simulink model "oppg1_system"  (R2014b)
settings: Solver=ode45  StartTime=0.0  StopTime=10  FixedStep=0.1  RelTol=1e-3
values from neighbouring files (symbols this model uses):
  A = 1    [main_1.m]    (also in main_tau.m)
  h_0 = 0    [main_1.m]    (also in main_tau.m)
  h_r = 0.5    [main_1.m]    (also in main_tau.m)
  k = 1    [main_1.m]    (also in main_tau.m)
  k_i = 0.1    [main_1.m]    (also in main_tau.m = 4)
  k_p = 100    [main_1.m]    (also in main_tau.m)
  rho = 1000    [main_1.m]    (also in main_tau.m)
  tau = 0    [main_1.m]    (also in main_tau.m = tau_list(i))
  w_f = 10    [main_1.m]    (also in main_tau.m = 0)
settings Model: Creator=rende_000  LastModifiedBy=rende_000

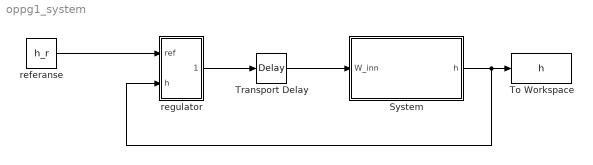
== system oppg1_system ==
  System : Subsystem
  To Workspace : ToWorkspace  VariableName=h  SaveFormat=Timeseries  SampleTime=-1
  Transport Delay : TransportDelay  DelayTime=tau
  referanse : Constant  Value=h_r
  regulator : Subsystem
  wires:
  System/1(h) -> regulator/2(h), To Workspace/1
  referanse/1 -> regulator/1(ref)
  regulator/1(Pådrag) -> Transport Delay/1
  Transport Delay/1 -> System/1(W_inn)

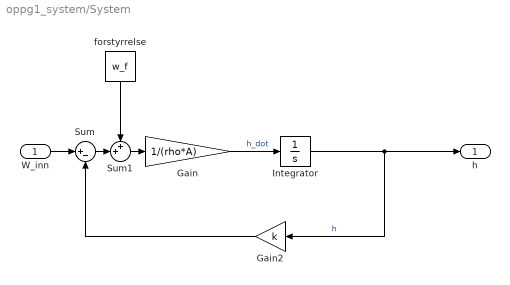
== system oppg1_system/System ==
  W_inn : Inport
  Gain : Gain  Gain=1/(rho*A)
  Gain2 : Gain  Gain=k
  Integrator : Integrator  InitialCondition=h_0
  Sum : Sum  Inputs=|+-
  Sum1 : Sum  Inputs=++|
  forstyrrelse : Constant  Value=w_f
  h : Outport
  wires:
  Gain2/1 -> Sum/2
  Integrator/1 -> h/1, Gain2/1  "h"
  Gain/1 -> Integrator/1  "h_dot"
  W_inn/1 -> Sum/1
  Sum1/1 -> Gain/1
  Sum/1 -> Sum1/2
  forstyrrelse/1 -> Sum1/1

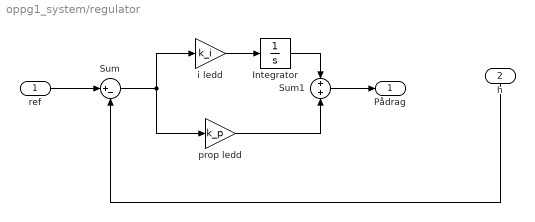
== system oppg1_system/regulator ==
  ref : Inport
  h : Inport  Port=2
  Integrator : Integrator
  Sum : Sum  Inputs=|+-
  Sum1 : Sum  Inputs=+|+
  i ledd : Gain  Gain=k_i
  prop ledd : Gain  Gain=k_p
  Pådrag : Outport
  wires:
  h/1 -> Sum/2
  ref/1 -> Sum/1
  Sum/1 -> i ledd/1, prop ledd/1
  Integrator/1 -> Sum1/1
  i ledd/1 -> Integrator/1
  Sum1/1 -> Pådrag/1
  prop ledd/1 -> Sum1/2
